simulink library "neural"  (Simulink 7.5)
settings: Solver=ode45  SolverMode=SingleTasking  StartTime=0.0  StopTime=10.0  RelTol=1e-3
undefined symbols (not defined in the file): sfunxy2
libraries: simulink x2
(part 1 of 2)
settings Model: Creator=mani  LastModifiedBy=mark  ExtModeAutoUpdateStatusClock=off

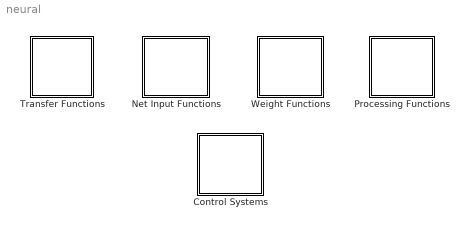
== system neural ==
  Control Systems : Subsystem
      mask Display:
      | e = 0.06;
      | c1 = [255 130 130]/255;
      | c2 = ([255 130 130]+0)/383;
      | c3 = ([255 130 130]+128)/383;
      | patch([0 1 1 0],[0 0 1 1],c1);
      | patch([0 1 1 1-e 1-e 0+e],[0 0 1 1-e 0+e 0+e],c2);
      | patch([0 0 1 1-e 0+e 0+e],[0 1 1 1-e 1-e 0+e],c3);
      | plot([0 1 1 0 0],[0 0 1 1 0])
      | disp('Control')
  Net Input Functions : Subsystem
      mask Display:
      | e = 0.06;
      | c1 = [255 130 130]/255;
      | c2 = ([255 130 130]+0)/383;
      | c3 = ([255 130 130]+128)/383;
      | patch([0 1 1 0],[0 0 1 1],c1);
      | patch([0 1 1 1-e 1-e 0+e],[0 0 1 1-e 0+e 0+e],c2);
      | patch([0 0 1 1-e 0+e 0+e],[0 1 1 1-e 1-e 0+e],c3);
      | plot([0 1 1 0 0],[0 0 1 1 0])
      | disp('N')
  Processing Functions : Subsystem
      mask Display:
      | e = 0.06;
      | c1 = [255 130 130]/255;
      | c2 = ([255 130 130]+0)/383;
      | c3 = ([255 130 130]+128)/383;
      | patch([0 1 1 0],[0 0 1 1],c1);
      | patch([0 1 1 1-e 1-e 0+e],[0 0 1 1-e 0+e 0+e],c2);
      | patch([0 0 1 1-e 0+e 0+e],[0 1 1 1-e 1-e 0+e],c3);
      | plot([0 1 1 0 0],[0 0 1 1 0])
      | disp('X<=>Y')
  Transfer Functions : Subsystem
      mask Display:
      | e = 0.06;
      | c1 = [255 130 130]/255;
      | c2 = ([255 130 130]+0)/383;
      | c3 = ([255 130 130]+128)/383;
      | patch([0 1 1 0],[0 0 1 1],c1);
      | patch([0 1 1 1-e 1-e 0+e],[0 0 1 1-e 0+e 0+e],c2);
      | patch([0 0 1 1-e 0+e 0+e],[0 1 1 1-e 1-e 0+e],c3);
      | color('white')
      | plot([-1 1]*0.35+0.5,[0 0]+0.5)
      | plot([0 0]+0.5,[-1 1]*0.35+0.5)
      | color('black')
      | xx = -1:0.01:1;
      | plot(xx*0.35+0.5,1./(1+exp(-5*xx))*0.7+0.15)
      | plot([0 1 1 0 0],[0 0 1 1 0])
  Weight Functions : Subsystem
      mask Display:
      | e = 0.06;
      | c1 = [255 130 130]/255;
      | c2 = ([255 130 130]+0)/383;
      | c3 = ([255 130 130]+128)/383;
      | patch([0 1 1 0],[0 0 1 1],c1);
      | patch([0 1 1 1-e 1-e 0+e],[0 0 1 1-e 0+e 0+e],c2);
      | patch([0 0 1 1-e 0+e 0+e],[0 1 1 1-e 1-e 0+e],c3);
      | plot([0 1 1 0 0],[0 0 1 1 0])
      | disp('W')

== system neural/Control Systems ==
  Model Reference Controller : Subsystem  mask(NN Model Reference Control){Nrc=, Nic=, Njc=, IW_y=, IW_u=, IW_r=, B1_c=, B2_c=, LW_c=, retraining_c=, max_i_int=, min_i_int=, max_r_int=, min_r_int=, Ts=, S1=, Ni=, Nj=, sim_file=, trainfun=trainlm, Use_validation=, Use_Testing=, Use_Inc_training=, Use_previous_weights=, max_i=, min_i=, max_r=, min_r=, sam_training=, sam_training_c=, epochs=, epochs_c=, minp=, maxp=, mint=, maxt=, Normalize=, IW=, LW1_2=, LW2_1=, B1=, B2=, S1c=, Limit_output=, min_output=, max_output=, Ref_file=}
      mask prompts: Ts "Sample time"; trainfun "Training function Identification"; Limit_output "Limit output"
      mask help: Neural network model reference controller. You first train a neural network model of the plant to be controlled. Then train the controller so that the plant output will follow the output of a reference model. Double-click the Model Reference Control block to begin the plant and controller training.
      mask init:
      | xl = [0   .53     .53     .92   .92   .53   .53  NaN ];
      | yl = [.95 .95 1.05 1.05 .3   .3   .95 NaN  ];
      | x2 = [0 .53    NaN .92 1.2  ];
      | y2 = [.39 .39   NaN .65 .65  ];
      | t=(0:24)/24*2*pi;
      | xs = .07*cos(t)+.9;
      | ys = .07*sin(t)+.75;
      | 
      | x1t=.03; y1t=.31;
      | x2t=.03; y2t=.8;
      | x3t=.77; y3t=.53;
      | x4t=.77; y4t=.44;
      | x5t=.45; y5t=.66;
      | x6t=.45; y6t=.55;
      | x7t=.45; y7t=.44;
      settings: OpenFcn=nncontrolutil('nnmodref','',gcbh,gcb,'');
      mask Help: helpview([docroot '/toolbox/nnet/control5.html']);
      mask StyleString: edit,edit,edit,edit,edit,edit,edit,edit,edit,edit,edit,edit,edit,edit,edit,edit,edit,edit,edit,popup(trainbfg|trainbr |traincgb|traincgf|traincgp|traingd|traingdm|traingda|traingdx|trainlm |trainoss|trainrp |trainscg),edit,edit,edit,edit,edit,edit,edit,edit,edit,edit,edit,edit,edit,edit,edit,edit,edit,edit,edit,edit,edit,edit,edit,edit,edit,edit,edit
      mask Display:
      | e = 0.06;
      | c1 = [120 150 230]/255;
      | c2 = ([120 150 230]+0)/383;
      | c3 = ([120 150 230]+128)/383;
      | patch([0 1 1 0],[0 0 1 1],c1);
      | patch([0 1 1 1-e 1-e 0+e],[0 0 1 1-e 0+e 0+e],c2);
      | patch([0 0 1 1-e 0+e 0+e],[0 1 1 1-e 1-e 0+e],c3);
      | plot([[xl NaN x2]*.9-.075 ], [[yl  NaN y2]*.9-.1 ]);
      | plot([0 1 1 0 0],[0 0 1 1 0]);
      | text(x1t,y1t,'Plant Output');
      | text(x2t,y2t,'Reference');
      | text(x3t,y3t,'Control');
      | text(x4t,y4t,'Signal');
      | text(x5t,y5t,'Neural');
      | text(x6t,y6t,'Network');
      | text(x7t,y7t,'Controller');
  NARMA-L2 Controller : Subsystem  mask(NARMA-L2 Controller){Normalize=, IW1_1=, IW3_2=, IW5_3=, LW2_1=, LW4_3=, LW5_4=, LW6_5=, LW6_2=, B1=, B2=, B3=, B4=, Limit_output=, min_output=, max_output=, Use_Previous_Weights=, Ts=, S1=, Ni=, Nj=, sim_file=, trainfun=trainlm, Use_validation=, Use_Testing=, max_i=, min_i=, max_i_int=, min_i_int=, sam_training=, epochs=, minp=, maxp=, mint=, maxt=}
      mask prompts: Ts "Sample time"; trainfun "Training function"
      mask help: NARMA-L2 Controller. You first train a neural network model of the plant to be controlled. The controller is a rearrangement of the trained plant model. Double-click the NARMA-L2 Controller block to begin the plant training.
      mask init:
      | xl = [0    .4   NaN  .33  .55   .55  .33  .33  NaN .80  .92 .92];
      | yl = [.95 .95 NaN  .75  .75   .55  .55  .75  NaN  .95 .95 .65];
      | x2 = [0    .43 NaN .45 .45    NaN .92 1.2 NaN .63 .85 .85 .63 .63 ];
      | y2 = [.39 .39 NaN  .41 .55   NaN .65 .65 NaN .75 .75  .55  .55  .75];
      | x3 = [.45 .45 NaN .42 .45 .48  NaN .33 .4 .33];
      | y3 = [.75 .90 NaN .83 .90 .83  NaN  .98 .95 .92];
      | x4 = [.75 .75 NaN .72 .75 .78  NaN  .5 .7 NaN .63 .7 .63];
      | y4 = [.75 .90 NaN .83 .90 .83  NaN .95 .95 NaN .98 .95 .92];
      | x5 = [.43 .43 .77 .77 .43 NaN .36 .43 .36 NaN .75 .75];
      | y5 = [.37 .41 .41 .37 .37 NaN .42 .39 .36 NaN .41 .55];
      | x6 = [.92 .92 .77 NaN .84 .77 .84];
      | y6 = [.65 .39 .39 NaN .42 .39 .36];
      | x1t=.03; y1t=.31;
      | x2t=.03; y2t=.85;
      | x8t=.03;y8t=.21;
      | x3t=.77; y3t=.53;
      | x4t=.77; y4t=.44;
      | x5t=.34; y5t=.49;
      | x6t=.58; y6t=.49;
      | 
      | 
      | t=(0:24)/24*2*pi;
      | xs = .05*cos(t);
      | ys = .05*sin(t);
      | xs1=xs+.45;
      | ys1=ys+.95;
      | xs2=xs+.75;
      | ys2=ys+.95;
      settings: OpenFcn=nncontrolutil('nnident','',gcbh,gcb,'narma_l2');
      mask Help: helpview([docroot '/toolbox/nnet/control4.html']);
      mask StyleString: edit,edit,edit,edit,edit,edit,edit,edit,edit,edit,edit,edit,edit,edit,edit,edit,edit,edit,edit,edit,edit,edit,popup(trainbfg|trainbr |traincgb|traincgf|traincgp|traingd|traingdm|traingda|traingdx|trainlm |trainoss|trainrp |trainscg),edit,edit,edit,edit,edit,edit,edit,edit,edit,edit,edit,edit
      mask Display:
      | e = 0.06;
      | c1 = [120 150 230]/255;
      | c2 = ([120 150 230]+0)/383;
      | c3 = ([120 150 230]+128)/383;
      | patch([0 1 1 0],[0 0 1 1],c1);
      | patch([0 1 1 1-e 1-e 0+e],[0 0 1 1-e 0+e 0+e],c2);
      | patch([0 0 1 1-e 0+e 0+e],[0 1 1 1-e 1-e 0+e],c3);
      | plot([[xl NaN x2]*.9-.075 ], [[yl  NaN y2]*.9-.1 ]);
      | plot([[xl NaN x2]*.9-.075 ], [[yl  NaN y2]*.9-.1 ]);
      | plot([[x3 NaN xs1 NaN xs2]*.9-.075 ], [[y3 NaN ys1 NaN ys2]*.9-.1 ]);
      | plot([x4 NaN x5]*.9-.075,[y4 NaN y5]*.9-.1);
      | plot([x6 NaN ]*.9-.075,[y6 NaN ]*.9-.1);
      | plot([0 1 1 0 0],[0 0 1 1 0]);
      | text(x1t,y1t,'Plant');
      | text(x8t,y8t,'Output');
      | text(x2t,y2t,'Reference');
      | text(x3t,y3t,'Control');
      | text(x4t,y4t,'Signal');
      | text(x5t,y5t,'f');
      | text(x6t,y6t,'g');
  NN Predictive Controller : Subsystem  mask(NN Predictive Controller){epochs=, minp=, maxp=, mint=, maxt=, Normalize=, IW=, LW1_2=, LW2_1=, B1=, B2=, max_i_int=, min_i_int=, limit_output=, max_output=, min_output=, Use_Previous_Weights=, N2=, Nu=, Ts=, rho=, alpha=, csrchfun=csrchbac, maxiter=, S1=, Ni=, Nj=, sim_file=, trainfun=trainlm, Use_validation=, Use_Testing=, max_i=, min_i=, sam_training=}
      mask prompts: Ts "Sample time"; rho "rho (typically = 0.03)"; alpha "alpha (typically = 0.001)"; csrchfun "Minimization rutine"; trainfun "Training function"
      mask help: NN Predictive Controller. You first train a neural network model of the plant to be controlled. The controller uses the plant model to predict plant performance over a specified time horizon. An optimization algorithm determines the control signal that optimizes plant performance over this horizon. Double click the NN Predictive Controller block to train the plant model and set the controller parameters.
      mask init:
      | xl = [0   .53   .53     .85   .85  .53  .53  NaN .85  .92 .92];
      | yl = [.95 .95 1.05  1.05   .82  .82  .95  NaN  .95 .95 .65];
      | x2 = [0 .53    NaN .92 1.2 NaN .53 .85 .85 .53 .53 ];
      | y2 = [.39 .39   NaN .65 .65 NaN .59 .59 .29 .29  .59];
      | x3 = [.67 .67 NaN .64 .67 .70 NaN .53 .4   .4   .53 NaN .46 .53 .46];
      | y3 = [.59 .82 NaN .66 .59 .66 NaN .55 .55 .86 .86 NaN  .89 .86 .83];
      | 
      | x1t=.03; y1t=.31;
      | x2t=.03; y2t=.8;
      | x8t=.03;y8t=.21;
      | x3t=.77; y3t=.53;
      | x4t=.77; y4t=.44;
      | x5t=.45; y5t=.76;
      | x6t=.45; y6t=.35;
      | x7t=.45; y7t=.25;
      settings: OpenFcn=nncontrolutil('nnpredict','',gcbh,gcb);
      mask Help: helpview([docroot '/toolbox/nnet/control3.html']);
      mask StyleString: edit,edit,edit,edit,edit,edit,edit,edit,edit,edit,edit,edit,edit,edit,edit,edit,edit,edit,edit,edit,edit,edit,popup(csrchgol|csrchbac|csrchhyb|csrchbre|csrchcha),edit,edit,edit,edit,edit,popup(trainbfg|trainbr |traincgb|traincgf|traincgp|traingd|traingdm|traingda|traingdx|trainlm |trainoss|trainrp |trainscg),edit,edit,edit,edit,edit
      mask Display:
      | e = 0.06;
      | c1 = [120 150 230]/255;
      | c2 = ([120 150 230]+0)/383;
      | c3 = ([120 150 230]+128)/383;
      | patch([0 1 1 0],[0 0 1 1],c1);
      | patch([0 1 1 1-e 1-e 0+e],[0 0 1 1-e 0+e 0+e],c2);
      | patch([0 0 1 1-e 0+e 0+e],[0 1 1 1-e 1-e 0+e],c3);
      | plot([[xl NaN x2]*.9-.075 ], [[yl  NaN y2]*.9-.1 ]);
      | plot([[xl NaN x2]*.9-.075 ], [[yl  NaN y2]*.9-.1 ]);
      | plot([[x3]*.9-.075 ], [[y3]*.9-.1 ]);
      | plot([0 1 1 0 0],[0 0 1 1 0]);
      | text(x1t,y1t,'Plant');
      | text(x8t,y8t,'Output');
      | text(x2t,y2t,'Reference');
      | text(x3t,y3t,'Control');
      | text(x4t,y4t,'Signal');
      | text(x5t,y5t,'Optim.');
      | text(x6t,y6t,'NN');
      | text(x7t,y7t,'Model');
  X(2Y)  Graph : Subsystem  LoadFcn=sfunxy2([],[],[],'LoadBlock')  StartFcn=sfunxy2([],[],[],'Start')  StopFcn=sfunxy2([],[],[],'Stop')  mask(X(2Y) scope.){xmin=0, xmax=5, ymin=21, ymax=22, st=-1}
      mask prompts: xmin "x-min:"; xmax "x-max:"; ymin "y-min:"; ymax "y-max:"; st "Sample time:"
      mask help: X(2Y) scope using MATLAB graph window. First input is used as time base. Enter plotting ranges.
      settings: CopyFcn=sfunxy2([],[],[],'CopyBlock')  DeleteFcn=sfunxy2([],[],[],'DeleteBlock')  NameChangeFcn=sfunxy2([],[],[],'NameChange')
      mask Help: This block can be used to explore limit cycles. Look at the m-file sfunxy.m to see how it works.
      mask Display:
      | e = 0.06;
      | c1 = [120 230 180]/255;
      | c2 = ([120 230 180]+0)/383;
      | c3 = ([120 230 180]+128)/383;
      | patch([0 1 1 0],[0 0 1 1],c1);
      | patch([0 1 1 1-e 1-e 0+e],[0 0 1 1-e 0+e 0+e],c2);
      | patch([0 0 1 1-e 0+e 0+e],[0 1 1 1-e 1-e 0+e],c3);
      | plot([0 1 1 0 0],[0 0 1 1 0]);
      | plot([.05 .95 .95 .05 .05],[.45 .45 .95 .95 .45], 0.5+cos(0:0.1:2*pi)*0.3,0.7+sin(0:0.1:2*pi)*0.2)

== system neural/Net Input Functions ==
  netprod : Product  OutDataType=sfix(16)  OutScaling=2^0  SaturateOnIntegerOverflow=on  RndMeth=Zero  InputSameDT=on  OutDataTypeStr=Inherit: Same as first input
  netsum : Sum  Inputs=2  OutDataType=sfix(16)  OutScaling=2^0  SaturateOnIntegerOverflow=on  InputSameDT=on  OutDataTypeStr=Inherit: Same as first input

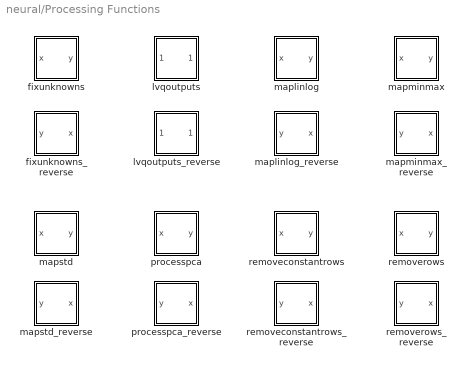
== system neural/Processing Functions ==
  fixunknowns : Subsystem  AncestorBlock=neural/Processing Functions/fixunknowns  mask(FIXUNKNOWNS Preprocess){inputSize=4, indices=[1 2 0 3 0 4]}
      mask prompts: inputSize "Input size"
      mask help: While Simulink does not allow the encoding of unknown values as NaN values, this block ensures networks which use FIXUNKNOWNS at the command line operate correctly in Simulink.
      mask Help: helpview([docroot '/toolbox/nnet/fixunknowns.html']);
      mask Display:
      | e = 0.06;
      | c1 = [120 150 230]/255;
      | c2 = ([120 150 230]+0)/383;
      | c3 = ([120 150 230]+128)/383;
      | patch([0 1 1 0],[0 0 1 1],c1);
      | patch([0 1 1 1-e 1-e 0+e],[0 0 1 1-e 0+e 0+e],c2);
      | patch([0 0 1 1-e 0+e 0+e],[0 1 1 1-e 1-e 0+e],c3);
      | plot([0 1 1 0 0],[0 0 1 1 0])
      | port_label('input',1,'x')
      | port_label('output',1,'y')
  fixunknowns_reverse : Subsystem  AncestorBlock=neural/Processing Functions/fixunknowns_reverse  mask(FIXUNKNOWNS Reverse Process){inputSize=6, indices=[1 2 4 6]}
      mask prompts: inputSize "Input size"
      mask help: While Simulink does not allow the encoding of unknown values as NaN values, this block ensures networks which use FIXUNKNOWNS at the command line operate correctly in Simulink.
      mask Help: helpview([docroot '/toolbox/nnet/fixunknowns.html']);
      mask Display:
      | e = 0.06;
      | c1 = [120 150 230]/255;
      | c2 = ([120 150 230]+0)/383;
      | c3 = ([120 150 230]+128)/383;
      | patch([0 1 1 0],[0 0 1 1],c1);
      | patch([0 1 1 1-e 1-e 0+e],[0 0 1 1-e 0+e 0+e],c2);
      | patch([0 0 1 1-e 0+e 0+e],[0 1 1 1-e 1-e 0+e],c3);
      | plot([0 1 1 0 0],[0 0 1 1 0])
      | port_label('input',1,'y')
      | port_label('output',1,'x')
  lvqoutputs : Subsystem
      mask Type: LVQOUTPUTS Preprocess
      mask Description: LVQ outputs preprocessing
      mask Help: helpview([docroot '/toolbox/nnet/lvqoutputs.html']);
      mask Display:
      | e = 0.06;
      | c1 = [120 150 230]/255;
      | c2 = ([120 150 230]+0)/383;
      | c3 = ([120 150 230]+128)/383;
      | patch([0 1 1 0],[0 0 1 1],c1);
      | patch([0 1 1 1-e 1-e 0+e],[0 0 1 1-e 0+e 0+e],c2);
      | patch([0 0 1 1-e 0+e 0+e],[0 1 1 1-e 1-e 0+e],c3);
      | plot([0 1 1 0 0],[0 0 1 1 0])
      | port_label('input',1,'x')
      | port_label('output',1,'y')
  lvqoutputs_reverse : Subsystem  AncestorBlock=neural/Processing Functions/lvqoutput
      mask Type: LVQOUTPUTS Reverse Process
      mask Description: LVQ outputs reverse processsing
      mask Help: helpview([docroot '/toolbox/nnet/lvqoutputs.html']);
      mask Display:
      | e = 0.06;
      | c1 = [120 150 230]/255;
      | c2 = ([120 150 230]+0)/383;
      | c3 = ([120 150 230]+128)/383;
      | patch([0 1 1 0],[0 0 1 1],c1);
      | patch([0 1 1 1-e 1-e 0+e],[0 0 1 1-e 0+e 0+e],c2);
      | patch([0 0 1 1-e 0+e 0+e],[0 1 1 1-e 1-e 0+e],c3);
      | plot([0 1 1 0 0],[0 0 1 1 0])
      | port_label('input',1,'y')
      | port_label('output',1,'x')
  maplinlog : Subsystem  AncestorBlock=neural/Processing Functions/mapminmax  mask(MAPLINLOG Preprocess){xmin=[0; -1; -2], xmax=[1; 1; 2], ymin=-1, ymax=+1}
      mask prompts: xmin "Minimum X (Nx1 column)"; xmax "Maximum X (Nx1 column)"; ymin "Minimum Y"; ymax "Maximum Y"
      mask help: Maps each element of x from linear values to log values.
      mask Help: helpview([docroot '/toolbox/nnet/maplinlog.html']);
      mask Display:
      | e = 0.06;
      | c1 = [120 150 230]/255;
      | c2 = ([120 150 230]+0)/383;
      | c3 = ([120 150 230]+128)/383;
      | patch([0 1 1 0],[0 0 1 1],c1);
      | patch([0 1 1 1-e 1-e 0+e],[0 0 1 1-e 0+e 0+e],c2);
      | patch([0 0 1 1-e 0+e 0+e],[0 1 1 1-e 1-e 0+e],c3);
      | plot([0 1 1 0 0],[0 0 1 1 0])
      | port_label('input',1,'x')
      | port_label('output',1,'y')
  maplinlog_reverse : Subsystem  AncestorBlock=neural/Processing Functions/mapminmax_reverse  mask(MAPLINLOG Reverse Process){xmin=[0; -1; -2], xmax=[1; 1; 2], ymin=-1, ymax=+1}
      mask prompts: xmin "Minimum X (Nx1 column)"; xmax "Maximum X (Nx1 column)"; ymin "Minimum Y"; ymax "Maximum Y"
      mask help: Maps log values to linear.
      mask Help: helpview([docroot '/toolbox/nnet/maplinlog.html']);
      mask Display:
      | e = 0.06;
      | c1 = [120 150 230]/255;
      | c2 = ([120 150 230]+0)/383;
      | c3 = ([120 150 230]+128)/383;
      | patch([0 1 1 0],[0 0 1 1],c1);
      | patch([0 1 1 1-e 1-e 0+e],[0 0 1 1-e 0+e 0+e],c2);
      | patch([0 0 1 1-e 0+e 0+e],[0 1 1 1-e 1-e 0+e],c3);
      | plot([0 1 1 0 0],[0 0 1 1 0])
      | port_label('input',1,'y')
      | port_label('output',1,'x')
  mapminmax : Subsystem  AncestorBlock=neural/Processing Functions/mapminmax  mask(MAPMINMAX Preprocess){xmin=[0; -1; -2], xmax=[1; 1; 2], ymin=-1, ymax=+1}
      mask prompts: xmin "Minimum X (Nx1 column)"; xmax "Maximum X (Nx1 column)"; ymin "Minimum Y"; ymax "Maximum Y"
      mask help: Maps each element of x from its respective [minimum,maximum] interval to a common [minimum,maximum] interval.
      mask Help: helpview([docroot '/toolbox/nnet/mapminmax.html']);
      mask Display:
      | e = 0.06;
      | c1 = [120 150 230]/255;
      | c2 = ([120 150 230]+0)/383;
      | c3 = ([120 150 230]+128)/383;
      | patch([0 1 1 0],[0 0 1 1],c1);
      | patch([0 1 1 1-e 1-e 0+e],[0 0 1 1-e 0+e 0+e],c2);
      | patch([0 0 1 1-e 0+e 0+e],[0 1 1 1-e 1-e 0+e],c3);
      | plot([0 1 1 0 0],[0 0 1 1 0])
      | port_label('input',1,'x')
      | port_label('output',1,'y')
  mapminmax_reverse : Subsystem  AncestorBlock=neural/Processing Functions/mapminmax_reverse  mask(MAPMINMAX Reverse Process){xmin=[0; -1; -2], xmax=[1; 1; 2], ymin=-1, ymax=+1}
      mask prompts: xmin "Minimum X (Nx1 column)"; xmax "Maximum X (Nx1 column)"; ymin "Minimum Y"; ymax "Maximum Y"
      mask help: Maps each element of y from a common [minimum,maximum] interval to its own respective [minimum,maximum] interval.
      mask Help: helpview([docroot '/toolbox/nnet/mapminmax.html']);
      mask Display:
      | e = 0.06;
      | c1 = [120 150 230]/255;
      | c2 = ([120 150 230]+0)/383;
      | c3 = ([120 150 230]+128)/383;
      | patch([0 1 1 0],[0 0 1 1],c1);
      | patch([0 1 1 1-e 1-e 0+e],[0 0 1 1-e 0+e 0+e],c2);
      | patch([0 0 1 1-e 0+e 0+e],[0 1 1 1-e 1-e 0+e],c3);
      | plot([0 1 1 0 0],[0 0 1 1 0])
      | port_label('input',1,'y')
      | port_label('output',1,'x')
  mapstd : Subsystem  AncestorBlock=neural/Processing Functions/mapstd  mask(MAPSTD Preprocess){xmean=[0; -1; -2], xstd=[1; 1; 2], ymean=-1, ystd=+1}
      mask prompts: xmean "X Mean (Nx1 column)"; xstd "X Standard Deviation (Nx1 column)"; ymean "Y Mean"; ystd "Y Standard Deviation"
      mask help: Maps each elements of x from its respective mean and standard deviation to a common mean and std.
      mask Help: helpview([docroot '/toolbox/nnet/mapstd.html']);
      mask Display:
      | e = 0.06;
      | c1 = [120 150 230]/255;
      | c2 = ([120 150 230]+0)/383;
      | c3 = ([120 150 230]+128)/383;
      | patch([0 1 1 0],[0 0 1 1],c1);
      | patch([0 1 1 1-e 1-e 0+e],[0 0 1 1-e 0+e 0+e],c2);
      | patch([0 0 1 1-e 0+e 0+e],[0 1 1 1-e 1-e 0+e],c3);
      | plot([0 1 1 0 0],[0 0 1 1 0])
      | port_label('input',1,'x')
      | port_label('output',1,'y')
  mapstd_reverse : Subsystem  AncestorBlock=neural/Processing Functions/mapstd_reverse  mask(MAPSTD Reverse Process){xmean=[0; -1; -2], xstd=[1; 1; 2], ymean=-1, ystd=+1}
      mask prompts: xmean "X Mean (Nx1 column)"; xstd "X Standard Deviation (Nx1 column)"; ymean "Y Mean"; ystd "Y Standard Deviation"
      mask help: Maps each element of y from a common mean and standard deviation to its own respective mean and standard deviation.
      mask Help: helpview([docroot '/toolbox/nnet/mapstd.html']);
      mask Display:
      | e = 0.06;
      | c1 = [120 150 230]/255;
      | c2 = ([120 150 230]+0)/383;
      | c3 = ([120 150 230]+128)/383;
      | patch([0 1 1 0],[0 0 1 1],c1);
      | patch([0 1 1 1-e 1-e 0+e],[0 0 1 1-e 0+e 0+e],c2);
      | patch([0 0 1 1-e 0+e 0+e],[0 1 1 1-e 1-e 0+e],c3);
      | plot([0 1 1 0 0],[0 0 1 1 0])
      | port_label('input',1,'y')
      | port_label('output',1,'x')
  processpca : Subsystem  AncestorBlock=neural/Processing Functions/removeconstantrows  mask(PROCESSPCA Process){transform=5}
      mask prompts: transform "Transform Matrix"
      mask help: Removes rows which were linearly dependent on other rows.
      mask Help: helpview([docroot '/toolbox/nnet/processpca.html']);
      mask Display:
      | e = 0.06;
      | c1 = [120 150 230]/255;
      | c2 = ([120 150 230]+0)/383;
      | c3 = ([120 150 230]+128)/383;
      | patch([0 1 1 0],[0 0 1 1],c1);
      | patch([0 1 1 1-e 1-e 0+e],[0 0 1 1-e 0+e 0+e],c2);
      | patch([0 0 1 1-e 0+e 0+e],[0 1 1 1-e 1-e 0+e],c3);
      | plot([0 1 1 0 0],[0 0 1 1 0])
      | port_label('input',1,'x')
      | port_label('output',1,'y')
  processpca_reverse : Subsystem  AncestorBlock=neural/Processing Functions/removeconstantrows_reverse  mask(PROCESSPCA Reverse Process){inverse_transform=3}
      mask prompts: inverse_transform "Inverse transform matrix"
      mask help: Replaces rows which were removed for being linearly dependent on other rows.
      mask Help: helpview([docroot '/toolbox/nnet/processpca.html']);
      mask Display:
      | e = 0.06;
      | c1 = [120 150 230]/255;
      | c2 = ([120 150 230]+0)/383;
      | c3 = ([120 150 230]+128)/383;
      | patch([0 1 1 0],[0 0 1 1],c1);
      | patch([0 1 1 1-e 1-e 0+e],[0 0 1 1-e 0+e 0+e],c2);
      | patch([0 0 1 1-e 0+e 0+e],[0 1 1 1-e 1-e 0+e],c3);
      | plot([0 1 1 0 0],[0 0 1 1 0])
      | port_label('input',1,'y')
      | port_label('output',1,'x')
  removeconstantrows : Subsystem  AncestorBlock=neural/Processing Functions/removeconstantrows  mask(REMOVECONSTANTROWS Process){inputSize=5, keep=[1 2 4]}
      mask prompts: inputSize "Input size"; keep "Keep Indices"
      mask help: Removes rows from a vector in positions where the values are always constant.
      mask Help: helpview([docroot '/toolbox/nnet/removeconstantrows.html']);
      mask Display:
      | e = 0.06;
      | c1 = [120 150 230]/255;
      | c2 = ([120 150 230]+0)/383;
      | c3 = ([120 150 230]+128)/383;
      | patch([0 1 1 0],[0 0 1 1],c1);
      | patch([0 1 1 1-e 1-e 0+e],[0 0 1 1-e 0+e 0+e],c2);
      | patch([0 0 1 1-e 0+e 0+e],[0 1 1 1-e 1-e 0+e],c3);
      | plot([0 1 1 0 0],[0 0 1 1 0])
      | port_label('input',1,'x')
      | port_label('output',1,'y')
  removeconstantrows_reverse : Subsystem  AncestorBlock=neural/Processing Functions/removeconstantrows_reverse  mask(REMOVECONSTANTROWS Reverse Process){inputSize=3, constants=[5 9], rearrange=[1 2 4 3 5]}
      mask prompts: inputSize "Input size"; constants "Constant values"; rearrange "Rearrange indices (positive indices for input elements, negative for constant elements)"
      mask help:
      | Expands a vector by inserting constant values into it where they have previously been removed.
      |
      | Indices should be positive where they come from the input y, and negative where they come from the constants.
      mask Help: helpview([docroot '/toolbox/nnet/removeconstantrows.html']);
      mask Display:
      | e = 0.06;
      | c1 = [120 150 230]/255;
      | c2 = ([120 150 230]+0)/383;
      | c3 = ([120 150 230]+128)/383;
      | patch([0 1 1 0],[0 0 1 1],c1);
      | patch([0 1 1 1-e 1-e 0+e],[0 0 1 1-e 0+e 0+e],c2);
      | patch([0 0 1 1-e 0+e 0+e],[0 1 1 1-e 1-e 0+e],c3);
      | plot([0 1 1 0 0],[0 0 1 1 0])
      | port_label('input',1,'y')
      | port_label('output',1,'x')
  removerows : Subsystem  AncestorBlock=neural/Processing Functions/removerows  mask(REMOVEROWS Process){inputSize=5, keep=[1 2 4]}
      mask prompts: inputSize "Input size"; keep "Keep Indices"
      mask help: Removes rows from a vector.
      mask Help: helpview([docroot '/toolbox/nnet/removerows.html']);
      mask Display:
      | e = 0.06;
      | c1 = [120 150 230]/255;
      | c2 = ([120 150 230]+0)/383;
      | c3 = ([120 150 230]+128)/383;
      | patch([0 1 1 0],[0 0 1 1],c1);
      | patch([0 1 1 1-e 1-e 0+e],[0 0 1 1-e 0+e 0+e],c2);
      | patch([0 0 1 1-e 0+e 0+e],[0 1 1 1-e 1-e 0+e],c3);
      | plot([0 1 1 0 0],[0 0 1 1 0])
      | port_label('input',1,'x')
      | port_label('output',1,'y')
  removerows_reverse : Subsystem  AncestorBlock=neural/Processing Functions/removerows_reverse  mask(REMOVEROWS Reverse Process){inputSize=3, rearrange=[1 2 0 0 3]}
      mask prompts: inputSize "Input size"; rearrange "Rearrange indices (0 in position of unknowns)"
      mask help: Expands a vector by inserting elements into it where they have previously been removed.
      mask Help: helpview([docroot '/toolbox/nnet/removerows.html']);
      mask Display:
      | e = 0.06;
      | c1 = [120 150 230]/255;
      | c2 = ([120 150 230]+0)/383;
      | c3 = ([120 150 230]+128)/383;
      | patch([0 1 1 0],[0 0 1 1],c1);
      | patch([0 1 1 1-e 1-e 0+e],[0 0 1 1-e 0+e 0+e],c2);
      | patch([0 0 1 1-e 0+e 0+e],[0 1 1 1-e 1-e 0+e],c3);
      | plot([0 1 1 0 0],[0 0 1 1 0])
      | port_label('input',1,'y')
      | port_label('output',1,'x')

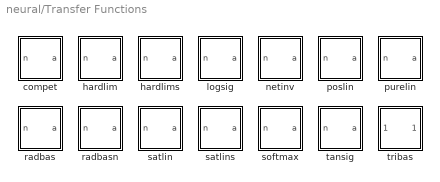
== system neural/Transfer Functions ==
  compet : Subsystem  AncestorBlock=neural/Transfer Functions/hardlim  mask(COMPET){layer_size=5}
      mask prompts: layer_size "Layer size"
      mask help: Competitive transfer function
      mask Help: helpview([docroot '/toolbox/nnet/compet.html']);
      mask Display:
      | e = 0.06;
      | c1 = [120 150 230]/255;
      | c2 = ([120 150 230]+0)/383;
      | c3 = ([120 150 230]+128)/383;
      | patch([0 1 1 0],[0 0 1 1],c1);
      | patch([0 1 1 1-e 1-e 0+e],[0 0 1 1-e 0+e 0+e],c2);
      | patch([0 0 1 1-e 0+e 0+e],[0 1 1 1-e 1-e 0+e],c3);
      | disp('C')
      | plot([0 1 1 0 0],[0 0 1 1 0]);
  hardlim : Subsystem
      mask Type: HARDLIM
      mask Description: Hard limit transfer function
      mask Help: helpview([docroot '/toolbox/nnet/hardlim.html']);
      mask Display:
      | e = 0.06;
      | c1 = [120 150 230]/255;
      | c2 = ([120 150 230]+0)/383;
      | c3 = ([120 150 230]+128)/383;
      | patch([0 1 1 0],[0 0 1 1],c1);
      | patch([0 1 1 1-e 1-e 0+e],[0 0 1 1-e 0+e 0+e],c2);
      | patch([0 0 1 1-e 0+e 0+e],[0 1 1 1-e 1-e 0+e],c3);
      | color('white')
      | plot([-1 1]*0.35+0.5,[0 0]+0.15)
      | color('black')
      | plot([-1 0 0 1]*0.35+0.5,[-1 -1 1 1]*0.35+0.5);
      | plot([0 1 1 0 0],[0 0 1 1 0]);
  hardlims : Subsystem
      mask Type: HARDLIMS
      mask Description: Symmetric hard limit transfer function
      mask Help: helpview([docroot '/toolbox/nnet/hardlims.html']);
      mask Display:
      | e = 0.06;
      | c1 = [120 150 230]/255;
      | c2 = ([120 150 230]+0)/383;
      | c3 = ([120 150 230]+128)/383;
      | patch([0 1 1 0],[0 0 1 1],c1);
      | patch([0 1 1 1-e 1-e 0+e],[0 0 1 1-e 0+e 0+e],c2);
      | patch([0 0 1 1-e 0+e 0+e],[0 1 1 1-e 1-e 0+e],c3);
      | color('white')
      | plot([-1 1]*0.35+0.5,[0 0]+0.5)
      | color('black')
      | plot([-1 0 0 1]*0.35+0.5,[-1 -1 1 1]*0.35+0.5);
      | plot([0 1 1 0 0],[0 0 1 1 0]);
  logsig : Subsystem
      mask Type: LOGSIG
      mask Description: Log sigmoid transfer function
      mask Help: helpview([docroot '/toolbox/nnet/logsig.html']);
      mask Display:
      | e = 0.06;
      | c1 = [120 150 230]/255;
      | c2 = ([120 150 230]+0)/383;
      | c3 = ([120 150 230]+128)/383;
      | patch([0 1 1 0],[0 0 1 1],c1);
      | patch([0 1 1 1-e 1-e 0+e],[0 0 1 1-e 0+e 0+e],c2);
      | patch([0 0 1 1-e 0+e 0+e],[0 1 1 1-e 1-e 0+e],c3);
      | color('white')
      | plot([0 1]*0.7+0.15,[0 0]+0.15);
      | plot([0 0]+0.5,[-1 1]*0.35+0.5);
      | color('black')
      | xx = [-1 -.9 -.8 -.7 -.6 -.5 -.4 -.3 -.2 -.1 0 .1 .2 .3 .4 .5 .6 .7 .8 .9 1];
      | yy = 1./(1+exp(-8*xx));
      | plot(xx*0.35+0.5,yy*0.7+0.15);
      | plot([0 1 1 0 0],[0 0 1 1 0]);
  netinv : Subsystem  AncestorBlock=neural/Transfer Functions/softmax
      mask Type: NETINV
      mask Description: Net inverse transfer function
      mask Help: helpview([docroot '/toolbox/nnet/netinv.html']);
      mask Display:
      | e = 0.06;
      | c1 = [120 150 230]/255;
      | c2 = ([120 150 230]+0)/383;
      | c3 = ([120 150 230]+128)/383;
      | patch([0 1 1 0],[0 0 1 1],c1);
      | patch([0 1 1 1-e 1-e 0+e],[0 0 1 1-e 0+e 0+e],c2);
      | patch([0 0 1 1-e 0+e 0+e],[0 1 1 1-e 1-e 0+e],c3);
      | disp('1/n')
      | plot([0 1 1 0 0],[0 0 1 1 0])
  poslin : Subsystem
      mask Type: POSLIN
      mask Description: Positive linear transfer function
      mask Help: helpview([docroot '/toolbox/nnet/poslin.html']);
      mask Display:
      | e = 0.06;
      | c1 = [120 150 230]/255;
      | c2 = ([120 150 230]+0)/383;
      | c3 = ([120 150 230]+128)/383;
      | patch([0 1 1 0],[0 0 1 1],c1);
      | patch([0 1 1 1-e 1-e 0+e],[0 0 1 1-e 0+e 0+e],c2);
      | patch([0 0 1 1-e 0+e 0+e],[0 1 1 1-e 1-e 0+e],c3);
      | color('white')
      | plot([-1 1]*0.35+0.5,[-1 -1]*0.35+0.5)
      | plot([0 0]+0.35,[-1 1]*0.35+0.5)
      | color('black')
      | plot([-1 -.5 1]*0.35+0.5,[-1 -1 1]*0.35+0.5)
      | plot([0 1 1 0 0],[0 0 1 1 0]);
  purelin : Subsystem
      mask Type: PURELIN
      mask Description: Linear transfer function
      mask Help: helpview([docroot '/toolbox/nnet/purelin.html']);
      mask Display:
      | e = 0.06;
      | c1 = [120 150 230]/255;
      | c2 = ([120 150 230]+0)/383;
      | c3 = ([120 150 230]+128)/383;
      | patch([0 1 1 0],[0 0 1 1],c1);
      | patch([0 1 1 1-e 1-e 0+e],[0 0 1 1-e 0+e 0+e],c2);
      | patch([0 0 1 1-e 0+e 0+e],[0 1 1 1-e 1-e 0+e],c3);
      | color('white')
      | plot([-1 1]*0.35+0.5,[0 0]+0.5)
      | plot([0 0]+0.5,[-1 1]*0.35+0.5)
      | color('black')
      | plot([-1 1]*0.35+0.5,[-1 1]*0.35+0.5)
      | plot([0 1 1 0 0],[0 0 1 1 0])
  radbas : Subsystem
      mask Type: RADBAS
      mask Description: Radial basis transfer function
      mask Help: helpview([docroot '/toolbox/nnet/radbas.html']);
      mask Display:
      | e = 0.06;
      | c1 = [120 150 230]/255;
      | c2 = ([120 150 230]+0)/383;
      | c3 = ([120 150 230]+128)/383;
      | patch([0 1 1 0],[0 0 1 1],c1);
      | patch([0 1 1 1-e 1-e 0+e],[0 0 1 1-e 0+e 0+e],c2);
      | patch([0 0 1 1-e 0+e 0+e],[0 1 1 1-e 1-e 0+e],c3);
      | color('white')
      | plot([-1 1]*0.35+0.5,[0 0]+0.15)
      | plot([0 0]+0.5,[0 1]*0.7+0.15)
      | color('black')
      | xx = -1:0.1:1;
      | plot(xx*0.35+0.5,exp(-4*(xx.^2))*0.8+0.1)
      | plot([0 1 1 0 0],[0 0 1 1 0])
  radbasn : Subsystem  AncestorBlock=neural/Transfer Functions/radbas
      mask Type: RADBASN
      mask Description: Normalized radial basis transfer function
      mask Help: helpview([docroot '/toolbox/nnet/radbasn.html']);
      mask Display:
      | e = 0.06;
      | c1 = [120 150 230]/255;
      | c2 = ([120 150 230]+0)/383;
      | c3 = ([120 150 230]+128)/383;
      | patch([0 1 1 0],[0 0 1 1],c1);
      | patch([0 1 1 1-e 1-e 0+e],[0 0 1 1-e 0+e 0+e],c2);
      | patch([0 0 1 1-e 0+e 0+e],[0 1 1 1-e 1-e 0+e],c3);
      | color('white')
      | plot([-1 1]*0.35+0.5,[0 0]+0.15)
      | plot([0 0]+0.5,[0 1]*0.7+0.15)
      | color('black')
      | xx = -1:0.1:1;
      | plot(xx*0.35+0.5,exp(-4*(xx.^2))*0.8+0.1)
      | plot([0 1 1 0 0],[0 0 1 1 0])
  satlin : Subsystem
      mask Type: SATLIN
      mask Description: Saturating linear transfer function
      mask Help: helpview([docroot '/toolbox/nnet/satlin.html']);
      mask Display:
      | e = 0.06;
      | c1 = [120 150 230]/255;
      | c2 = ([120 150 230]+0)/383;
      | c3 = ([120 150 230]+128)/383;
      | patch([0 1 1 0],[0 0 1 1],c1);
      | patch([0 1 1 1-e 1-e 0+e],[0 0 1 1-e 0+e 0+e],c2);
      | patch([0 0 1 1-e 0+e 0+e],[0 1 1 1-e 1-e 0+e],c3);
      | color('white')
      | plot([-1 1]*0.35+0.5,[0 0]+0.15)
      | plot(-[0.5 0.5]*0.35+0.5,[-1 1]*0.35+0.5)
      | color('black')
      | plot([-1 -0.5 0.5 1]*0.35+0.5,[-1 -1 1 1]*0.35+0.5)
      | plot([0 1 1 0 0],[0 0 1 1 0])
  satlins : Subsystem
      mask Type: SATLINS
      mask Description: Symmetric saturating linear transfer function
      mask Help: helpview([docroot '/toolbox/nnet/satlins.html']);
      mask Display:
      | e = 0.06;
      | c1 = [120 150 230]/255;
      | c2 = ([120 150 230]+0)/383;
      | c3 = ([120 150 230]+128)/383;
      | patch([0 1 1 0],[0 0 1 1],c1);
      | patch([0 1 1 1-e 1-e 0+e],[0 0 1 1-e 0+e 0+e],c2);
      | patch([0 0 1 1-e 0+e 0+e],[0 1 1 1-e 1-e 0+e],c3);
      | color('white')
      | plot([-1 1]*0.35+0.5,[0 0]+0.5)
      | plot([0 0]+0.5,[-1 1]*0.35+0.5)
      | color('black')
      | plot([-1 -0.5 0.5 1]*0.35+0.5,[-1 -1 1 1]*0.35+0.5)
      | plot([0 1 1 0 0],[0 0 1 1 0])
  softmax : Subsystem
      mask Type: SOFTMAX
      mask Description: Soft competitive transfer function
      mask Help: helpview([docroot '/toolbox/nnet/softmax.html']);
      mask Display:
      | e = 0.06;
      | c1 = [120 150 230]/255;
      | c2 = ([120 150 230]+0)/383;
      | c3 = ([120 150 230]+128)/383;
      | patch([0 1 1 0],[0 0 1 1],c1);
      | patch([0 1 1 1-e 1-e 0+e],[0 0 1 1-e 0+e 0+e],c2);
      | patch([0 0 1 1-e 0+e 0+e],[0 1 1 1-e 1-e 0+e],c3);
      | disp('S')
      | plot([0 1 1 0 0],[0 0 1 1 0])
  tansig : Subsystem
      mask Type: TANSIG
      mask Description: Symmetric sigmoid transfer function
      mask Help: helpview([docroot '/toolbox/nnet/tansig.html']);
      mask Display:
      | e = 0.06;
      | c1 = [120 150 230]/255;
      | c2 = ([120 150 230]+0)/383;
      | c3 = ([120 150 230]+128)/383;
      | patch([0 1 1 0],[0 0 1 1],c1);
      | patch([0 1 1 1-e 1-e 0+e],[0 0 1 1-e 0+e 0+e],c2);
      | patch([0 0 1 1-e 0+e 0+e],[0 1 1 1-e 1-e 0+e],c3);
      | color('white')
      | plot([-1 1]*0.35+0.5,[0 0]+0.5)
      | plot([0 0]+0.5,[-1 1]*0.35+0.5)
      | color('black')
      | xx = -1:0.01:1;
      | plot(xx*0.35+0.5,1./(1+exp(-5*xx))*0.7+0.15)
      | plot([0 1 1 0 0],[0 0 1 1 0])
  tribas : Subsystem
      mask Type: TRIBAS
      mask Description: Triangular basis transfer function
      mask Help: helpview([docroot '/toolbox/nnet/tribas.html']);
      mask Display:
      | e = 0.06;
      | c1 = [120 150 230]/255;
      | c2 = ([120 150 230]+0)/383;
      | c3 = ([120 150 230]+128)/383;
      | patch([0 1 1 0],[0 0 1 1],c1);
      | patch([0 1 1 1-e 1-e 0+e],[0 0 1 1-e 0+e 0+e],c2);
      | patch([0 0 1 1-e 0+e 0+e],[0 1 1 1-e 1-e 0+e],c3);
      | color('white')
      | plot([-1 1]*0.35+0.5,[0 0]+0.15)
      | plot([0 0]+0.5,[-1 1]*0.35+0.5)
      | color('black')
      | plot([-1 -.6 0 .6 1]*0.35+0.5,[0 0 1 0 0]*0.7+0.15)
      | plot([0 1 1 0 0],[0 0 1 1 0])

== system neural/Weight Functions ==
  dist : Subsystem
      mask Type: DIST
      mask Description: Euclidean distance weight function
      mask Help: helpview([docroot '/toolbox/nnet/dist.html']);
      mask Display:
      | e = 0.06;
      | c1 = [120 150 230]/255;
      | c2 = ([120 150 230]+0)/383;
      | c3 = ([120 150 230]+128)/383;
      | patch([0 1 1 0],[0 0 1 1],c1);
      | patch([0 1 1 1-e 1-e 0+e],[0 0 1 1-e 0+e 0+e],c2);
      | patch([0 0 1 1-e 0+e 0+e],[0 1 1 1-e 1-e 0+e],c3);
      | plot([0 1 1 0 0],[0 0 1 1 0])
      | port_label('input',1,'w')
      | port_label('input',2,'p')
      | port_label('output',1,'z')
  dotprod : Subsystem
      mask Type: DOTPROD
      mask Description: Dot product weight function
      mask Help: helpview([docroot '/toolbox/nnet/dotprod.html']);
      mask Display:
      | e = 0.06;
      | c1 = [120 150 230]/255;
      | c2 = ([120 150 230]+0)/383;
      | c3 = ([120 150 230]+128)/383;
      | patch([0 1 1 0],[0 0 1 1],c1);
      | patch([0 1 1 1-e 1-e 0+e],[0 0 1 1-e 0+e 0+e],c2);
      | patch([0 0 1 1-e 0+e 0+e],[0 1 1 1-e 1-e 0+e],c3);
      | plot([0 1 1 0 0],[0 0 1 1 0])
      | port_label('input',1,'w')
      | port_label('input',2,'p')
      | port_label('output',1,'z')
  negdist : Subsystem
      mask Type: NEGDIST
      mask Description: Negative euclidean distance weight function
      mask Help: helpview([docroot '/toolbox/nnet/negdist.html']);
      mask Display:
      | e = 0.06;
      | c1 = [120 150 230]/255;
      | c2 = ([120 150 230]+0)/383;
      | c3 = ([120 150 230]+128)/383;
      | patch([0 1 1 0],[0 0 1 1],c1);
      | patch([0 1 1 1-e 1-e 0+e],[0 0 1 1-e 0+e 0+e],c2);
      | patch([0 0 1 1-e 0+e 0+e],[0 1 1 1-e 1-e 0+e],c3);
      | plot([0 1 1 0 0],[0 0 1 1 0])
      | port_label('input',1,'w')
      | port_label('input',2,'p')
      | port_label('output',1,'z')
  normprod : Subsystem
      mask Type: NORMPROD
      mask Description: Normalized dot product weight function
      mask Help: helpview([docroot '/toolbox/nnet/normprod.html']);
      mask Display:
      | e = 0.06;
      | c1 = [120 150 230]/255;
      | c2 = ([120 150 230]+0)/383;
      | c3 = ([120 150 230]+128)/383;
      | patch([0 1 1 0],[0 0 1 1],c1);
      | patch([0 1 1 1-e 1-e 0+e],[0 0 1 1-e 0+e 0+e],c2);
      | patch([0 0 1 1-e 0+e 0+e],[0 1 1 1-e 1-e 0+e],c3);
      | plot([0 1 1 0 0],[0 0 1 1 0])
      | port_label('input',1,'w')
      | port_label('input',2,'p')
      | port_label('output',1,'z')

== system neural/Control Systems/Model Reference Controller ==
  Reference : Inport  OutDataType=sfix(16)  OutScaling=2^0
  Plant Output : Inport  Port=2  OutDataType=sfix(16)  OutScaling=2^0
  NN Controller : Subsystem
  NN Plant : Subsystem
  Terminator : Terminator
  Terminator1 : Terminator
  Control Signal : Outport  OutDataType=sfix(16)  OutScaling=2^0
  wires:
  NN Plant/2(yhat1) -> Terminator1/1
  NN Plant/1(yhat) -> Terminator/1
  Reference/1 -> NN Controller/1(r)
  NN Controller/1(uhat) -> NN Controller/2(u), Control Signal/1, NN Plant/1(u)
  Plant Output/1 -> NN Controller/3(y), NN Plant/2(y)

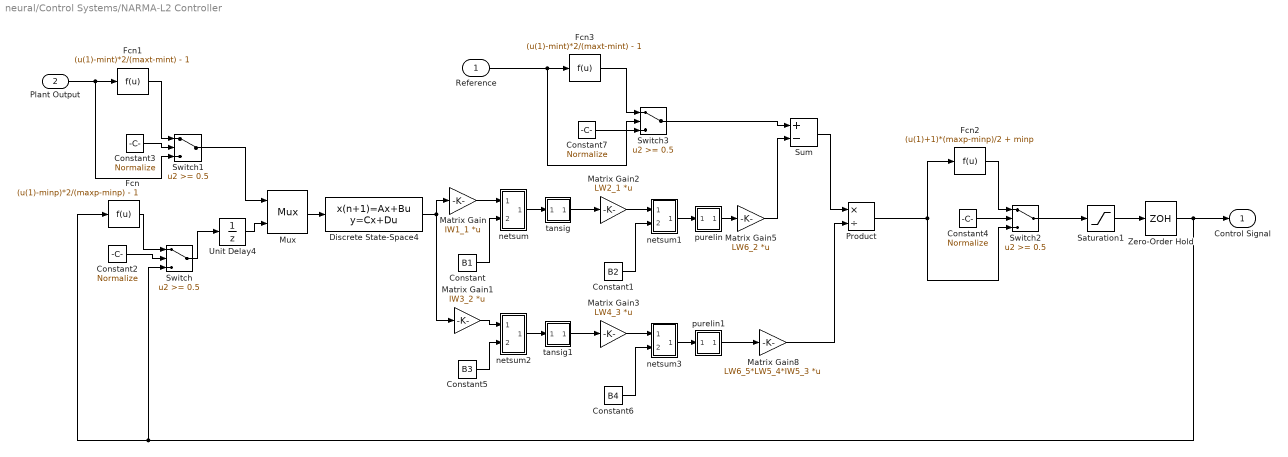
== system neural/Control Systems/NARMA-L2 Controller ==
  Reference : Inport  OutDataType=sfix(16)  OutScaling=2^0
  Plant Output : Inport  Port=2  OutDataType=sfix(16)  OutScaling=2^0
  Constant : Constant  Value=B1  OutDataType=sfix(16)  OutScaling=2^0
  Constant1 : Constant  Value=B2  OutDataType=sfix(16)  OutScaling=2^0
  Constant{2..4,7} (4 alike) : Constant  Value=Normalize  OutDataType=sfix(16)  OutScaling=2^0
  Constant5 : Constant  Value=B3  OutDataType=sfix(16)  OutScaling=2^0
  Constant6 : Constant  Value=B4  OutDataType=sfix(16)  OutScaling=2^0
  Discrete State-Space4 : DiscreteStateSpace  A=blkdiag([zeros(1,Nj-1);eye(Nj-2,Nj-2) zeros(Nj-2,1)],[zeros(1,Ni-1);eye(Ni-2,Ni-2) zeros(Ni-2,1)])  B=blkdiag(eye(Nj-1,1),eye(Ni-1,1))  C=blkdiag([zeros(1,Nj-1);eye(Nj-1,Nj-1)],[zeros(eye(double(Ni>1)),Ni-1);eye(Ni-2,Ni-1)])  D=blkdiag([1;zeros(Nj-1,1)],[eye(double(Ni>1));zeros(Ni-2,1)])  SampleTime=Ts
  Fcn : Fcn  Expr=(u(1)-minp)*2/(maxp-minp) - 1
  Fcn1 : Fcn  Expr=(u(1)-mint)*2/(maxt-mint) - 1
  Fcn2 : Fcn  Expr=(u(1)+1)*(maxp-minp)/2 + minp
  Fcn3 : Fcn  Expr=(u(1)-mint)*2/(maxt-mint) - 1
  Matrix Gain : Gain  Gain=IW1_1  Multiplication=Matrix(K*u)  ParameterDataType=sfix(16)  ParameterScaling=2^0  OutDataType=sfix(16)  OutScaling=2^0  SaturateOnIntegerOverflow=on  OutDataTypeStr=Inherit: Same as input  ParamDataTypeStr=Inherit: Same as input
  Matrix Gain1 : Gain  Gain=IW3_2  Multiplication=Matrix(K*u)  ParameterDataType=sfix(16)  ParameterScaling=2^0  OutDataType=sfix(16)  OutScaling=2^0  SaturateOnIntegerOverflow=on  OutDataTypeStr=Inherit: Same as input  ParamDataTypeStr=Inherit: Same as input
  Matrix Gain2 : Gain  Gain=LW2_1  Multiplication=Matrix(K*u)  ParameterDataType=sfix(16)  ParameterScaling=2^0  OutDataType=sfix(16)  OutScaling=2^0  SaturateOnIntegerOverflow=on  OutDataTypeStr=Inherit: Same as input  ParamDataTypeStr=Inherit: Same as input
  Matrix Gain3 : Gain  Gain=LW4_3  Multiplication=Matrix(K*u)  ParameterDataType=sfix(16)  ParameterScaling=2^0  OutDataType=sfix(16)  OutScaling=2^0  SaturateOnIntegerOverflow=on  OutDataTypeStr=Inherit: Same as input  ParamDataTypeStr=Inherit: Same as input
  Matrix Gain5 : Gain  Gain=LW6_2  Multiplication=Matrix(K*u)  ParameterDataType=sfix(16)  ParameterScaling=2^0  OutDataType=sfix(16)  OutScaling=2^0  SaturateOnIntegerOverflow=on  OutDataTypeStr=Inherit: Same as input  ParamDataTypeStr=Inherit: Same as input
  Matrix Gain8 : Gain  Gain=LW6_5*LW5_4*IW5_3  Multiplication=Matrix(K*u)  ParameterDataType=sfix(16)  ParameterScaling=2^0  OutDataType=sfix(16)  OutScaling=2^0  SaturateOnIntegerOverflow=on  OutDataTypeStr=Inherit: Same as input  ParamDataTypeStr=Inherit: Same as input
  Mux : Mux  Inputs=2
      settings: DisplayOption=signals
  Product : Product  Inputs=*/  OutDataType=sfix(16)  OutScaling=2^0  SaturateOnIntegerOverflow=on  RndMeth=Zero  InputSameDT=on  OutDataTypeStr=Inherit: Same as first input
  Saturation1 : Saturate  UpperLimit=max_i  LowerLimit=min_i
  Sum : Sum  Inputs=+-  OutDataType=sfix(16)  OutScaling=2^0  SaturateOnIntegerOverflow=on  InputSameDT=on  OutDataTypeStr=Inherit: Same as first input
  Switch{,1..3} (4 alike) : Switch  Threshold=0.5  SaturateOnIntegerOverflow=on  InputSameDT=on
  Unit Delay4 : UnitDelay  SampleTime=Ts
  Zero-Order Hold : ZeroOrderHold  SampleTime=Ts
  netsum : Subsystem
      mask Display: disp('+')
  netsum1 : Subsystem
      mask Display: disp('+')
  netsum2 : Subsystem
      mask Display: disp('+')
  netsum3 : Subsystem
      mask Display: disp('+')
  purelin : Subsystem
      mask Display: plot([-1 1],[0 0],[-1 1],[-1 1])
  purelin1 : Subsystem
      mask Display: plot([-1 1],[0 0],[-1 1],[-1 1])
  tansig : Subsystem
      mask Display: plot([-1 1],[0 0],[-1 -.9 -.8 -.7 -.6 -.5 -.4 -.3 -.2 -.1 0 .1 .2 .3 .4 .5 .6 .7 .8 .9 1],2./(1+exp(-8*[-1 -.9 -.8 -.7 -.6 -.5 -.4 -.3 -.2 -.1 0 .1 .2 .3 .4 .5 .6 .7 .8 .9 1]))-1)
  tansig1 : Subsystem
      mask Display: plot([-1 1],[0 0],[-1 -.9 -.8 -.7 -.6 -.5 -.4 -.3 -.2 -.1 0 .1 .2 .3 .4 .5 .6 .7 .8 .9 1],2./(1+exp(-8*[-1 -.9 -.8 -.7 -.6 -.5 -.4 -.3 -.2 -.1 0 .1 .2 .3 .4 .5 .6 .7 .8 .9 1]))-1)
  Control Signal : Outport  OutDataType=sfix(16)  OutScaling=2^0
  wires:
  Saturation1/1 -> Zero-Order Hold/1
  Switch/1 -> Unit Delay4/1
  Unit Delay4/1 -> Mux/2
  Constant2/1 -> Switch/2
  Fcn/1 -> Switch/1
  Zero-Order Hold/1 -> Switch/3, Fcn/1, Control Signal/1
  Discrete State-Space4/1 -> Matrix Gain1/1, Matrix Gain/1
  Mux/1 -> Discrete State-Space4/1
  Switch1/1 -> Mux/1
  Switch3/1 -> Sum/1
  Reference/1 -> Switch3/3, Fcn3/1
  Fcn3/1 -> Switch3/1
  Constant7/1 -> Switch3/2
  Matrix Gain8/1 -> Product/2
  purelin1/1(a) -> Matrix Gain8/1
  Sum/1 -> Product/1
  Matrix Gain5/1 -> Sum/2
  purelin/1(a) -> Matrix Gain5/1
  Matrix Gain1/1 -> netsum2/1(In1)
  tansig1/1(a) -> Matrix Gain3/1
  Constant5/1 -> netsum2/2(In2)
  netsum2/1(Out1) -> tansig1/1(n)
  Matrix Gain3/1 -> netsum3/1(In1)
  Constant6/1 -> netsum3/2(In2)
  netsum3/1(Out1) -> purelin1/1(n)
  Matrix Gain/1 -> netsum/1(In1)
  tansig/1(a) -> Matrix Gain2/1
  Constant/1 -> netsum/2(In2)
  netsum/1(Out1) -> tansig/1(n)
  Matrix Gain2/1 -> netsum1/1(In1)
  Constant1/1 -> netsum1/2(In2)
  netsum1/1(Out1) -> purelin/1(n)
  Plant Output/1 -> Switch1/3, Fcn1/1
  Fcn1/1 -> Switch1/1
  Constant3/1 -> Switch1/2
  Product/1 -> Fcn2/1, Switch2/3
  Constant4/1 -> Switch2/2
  Switch2/1 -> Saturation1/1
  Fcn2/1 -> Switch2/1

== system neural/Control Systems/NN Predictive Controller ==
  Reference : Inport  OutDataType=sfix(16)  OutScaling=2^0
  Plant output : Inport  Port=2  OutDataType=sfix(16)  OutScaling=2^0
  Mux : Mux
      settings: DisplayOption=signals
  NN model : Subsystem
  S-Function : S-Function  FunctionName=predopt  Parameters=N2,Ts,Nu,maxiter,csrchfun,rho,alpha,S1,IW,LW1_2,LW2_1,B1,B2,Ni,Nj,min_i,max_i,minp,maxp,mint,maxt,Normalize  EnableBusSupport=off
  Control Signal : Outport  OutDataType=sfix(16)  OutScaling=2^0
  wires:
  Plant output/1 -> Mux/2, NN model/2(y)
  Reference/1 -> Mux/1
  NN model/1(yhat) -> Mux/3
  NN model/2(yhat1) -> Mux/4
  S-Function/1 -> Control Signal/1, NN model/1(u)
  Mux/1 -> S-Function/1

== system neural/Control Systems/X(2Y)  Graph ==
  x : Inport  OutDataType=sfix(16)  OutScaling=2^0
  y1 : Inport  Port=2  OutDataType=sfix(16)  OutScaling=2^0
  y2 : Inport  Port=3  OutDataType=sfix(16)  OutScaling=2^0
  Mux : Mux  Inputs=3
  sfunxy : S-Function  FunctionName=sfunxy2  Parameters=[xmin xmax ymin ymax], st  EnableBusSupport=off
  wires:
  y2/1 -> Mux/3
  y1/1 -> Mux/2
  x/1 -> Mux/1
  Mux/1 -> sfunxy/1

== system neural/Processing Functions/fixunknowns ==
  x : Inport  OutDataType=sfix(16)  OutScaling=2^0
  Constants : Constant  OutDataType=sfix(16)  OutScaling=2^0
  Mux : Mux  Inputs=2
  Selector : Selector  IndexMode=Zero-based  InputPortWidth=inputSize+1  IndexOptions=Index vector (dialog)  Indices=indices  OutputSizes=1
  y : Outport  OutDataType=sfix(16)  OutScaling=2^0
  wires:
  Constants/1 -> Mux/1
  x/1 -> Mux/2
  Mux/1 -> Selector/1
  Selector/1 -> y/1

== system neural/Processing Functions/fixunknowns_reverse ==
  y : Inport  OutDataType=sfix(16)  OutScaling=2^0
  Selector : Selector  InputPortWidth=inputSize  IndexOptions=Index vector (dialog)  Indices=indices  OutputSizes=1
  x : Outport  OutDataType=sfix(16)  OutScaling=2^0
  wires:
  y/1 -> Selector/1
  Selector/1 -> x/1

== system neural/Processing Functions/lvqoutputs ==
  In1 : Inport
  Out1 : Outport
  wires:
  In1/1 -> Out1/1

== system neural/Processing Functions/lvqoutputs_reverse ==
  In1 : Inport
  Out1 : Outport
  wires:
  In1/1 -> Out1/1

== system neural/Processing Functions/maplinlog ==
  x : Inport  OutDataType=sfix(16)  OutScaling=2^0
  Add min y : Bias  Bias=ymin
  Subtract min x : Bias  Bias=-xmin
  range y / range x : Gain  Gain=(ymax-ymin)./(xmax-xmin)  ParameterDataType=sfix(16)  ParameterScaling=2^0  OutDataType=sfix(16)  OutScaling=2^0
  y : Outport  OutDataType=sfix(16)  OutScaling=2^0
  wires:
  Add min y/1 -> y/1
  range y / range x/1 -> Add min y/1
  Subtract min x/1 -> range y / range x/1
  x/1 -> Subtract min x/1

== system neural/Processing Functions/maplinlog_reverse ==
  y : Inport  OutDataType=sfix(16)  OutScaling=2^0
  Add min x : Bias  Bias=xmin
  Divide by range y : Gain  Gain=(xmax-xmin)./(ymax-ymin)  ParameterDataType=sfix(16)  ParameterScaling=2^0  OutDataType=sfix(16)  OutScaling=2^0
  Subtract min y : Bias  Bias=-ymin
  x : Outport  OutDataType=sfix(16)  OutScaling=2^0
  wires:
  y/1 -> Subtract min y/1
  Subtract min y/1 -> Divide by range y/1
  Divide by range y/1 -> Add min x/1
  Add min x/1 -> x/1

== system neural/Processing Functions/mapminmax ==
  x : Inport  OutDataType=sfix(16)  OutScaling=2^0
  Add min y : Bias  Bias=ymin
  Subtract min x : Bias  Bias=-xmin
  range y / range x : Gain  Gain=(ymax-ymin)./(xmax-xmin)  ParameterDataType=sfix(16)  ParameterScaling=2^0  OutDataType=sfix(16)  OutScaling=2^0
  y : Outport  OutDataType=sfix(16)  OutScaling=2^0
  wires:
  x/1 -> Subtract min x/1
  Subtract min x/1 -> range y / range x/1
  range y / range x/1 -> Add min y/1
  Add min y/1 -> y/1

== system neural/Processing Functions/mapminmax_reverse ==
  y : Inport  OutDataType=sfix(16)  OutScaling=2^0
  Add min x : Bias  Bias=xmin
  Divide by range y : Gain  Gain=(xmax-xmin)./(ymax-ymin)  ParameterDataType=sfix(16)  ParameterScaling=2^0  OutDataType=sfix(16)  OutScaling=2^0
  Subtract min y : Bias  Bias=-ymin
  x : Outport  OutDataType=sfix(16)  OutScaling=2^0
  wires:
  Add min x/1 -> x/1
  Divide by range y/1 -> Add min x/1
  Subtract min y/1 -> Divide by range y/1
  y/1 -> Subtract min y/1

== system neural/Processing Functions/mapstd ==
  x : Inport  OutDataType=sfix(16)  OutScaling=2^0
  Add y mean : Bias  Bias=ymean
  Subtract x mean : Bias  Bias=-xmean
  y std / x std : Gain  Gain=ystd./xstd  ParameterDataType=sfix(16)  ParameterScaling=2^0  OutDataType=sfix(16)  OutScaling=2^0
  y : Outport  OutDataType=sfix(16)  OutScaling=2^0
  wires:
  Add y mean/1 -> y/1
  y std / x std/1 -> Add y mean/1
  x/1 -> Subtract x mean/1
  Subtract x mean/1 -> y std / x std/1

== system neural/Processing Functions/mapstd_reverse ==
  y : Inport  OutDataType=sfix(16)  OutScaling=2^0
  Add x mean : Bias  Bias=xmean
  Subtract y mean : Bias  Bias=-ymean
  x std / y std : Gain  Gain=xstd./ystd  ParameterDataType=sfix(16)  ParameterScaling=2^0  OutDataType=sfix(16)  OutScaling=2^0
  x : Outport  OutDataType=sfix(16)  OutScaling=2^0
  wires:
  y/1 -> Subtract y mean/1
  Subtract y mean/1 -> x std / y std/1
  x std / y std/1 -> Add x mean/1
  Add x mean/1 -> x/1

== system neural/Processing Functions/processpca ==
  x : Inport  OutDataType=sfix(16)  OutScaling=2^0
  Constant1 : Constant  Value=transform  VectorParams1D=off  OutDataType=sfix(16)  OutScaling=2^0
  Product : Product  Multiplication=Matrix(*)  OutDataType=sfix(16)  OutScaling=2^0  RndMeth=Zero
  y : Outport  OutDataType=sfix(16)  OutScaling=2^0
  wires:
  Constant1/1 -> Product/1
  x/1 -> Product/2
  Product/1 -> y/1
